simulink model "crazyflie"  (R2023a)
settings: Solver=FixedStepDiscrete  StartTime=0.0  StopTime=160  FixedStep=0.001  RelTol=1e-3
undefined symbols (not defined in the file or in its folder): K
settings Model: PauseTimes=7  Creator=Zrean  LastModifiedBy=mosta
settings SolverCC: AlgebraicLoopSolver=TrustRegion
settings DataIOCC: ReturnWorkspaceOutputs=off
settings OptimizationCC: DefaultParameterBehavior=Inlined  UseDivisionForNetSlopeComputation=on  UseFloatMulNetSlope=on  UseSpecifiedMinMax=on  InlineInvariantSignals=on  PassReuseOutputArgsAs=Individual arguments  ZeroExternalMemoryAtStartup=off  ZeroInternalMemoryAtStartup=off  NoFixptDivByZeroProtection=on  EfficientFloat2IntCast=on  LifeSpan=1  EfficientTunableParamExpr=on
settings DebuggingCC: AlgebraicLoopMsg=error  ParameterTunabilityLossMsg=error  UnconnectedInputMsg=warning  UnconnectedOutputMsg=warning  UnconnectedLineMsg=warning  ArithmeticOperatorsInVariantConditions=warning
settings HardwareCC: ProdBitPerPointer=32  ProdBitPerSizeT=32  ProdBitPerPtrDiffT=32  ProdLargestAtomicInteger=Long  ProdLargestAtomicFloat=Double  ProdWordSize=32  ProdHWDeviceType=ARM Compatible->ARM Cortex
settings ModelReferenceCC: EnableRefExpFcnMdlSchedulingChecks=on
settings SFSimCC: SimUseLocalCustomCode=off  MATLABDynamicMemAlloc=off  CustomCodeUndefinedFunction=UseInterfaceOnly
settings RTWCC: Description=Embedded Coder  SystemTargetFile=ert.tlc  GenCodeOnly=on  TemplateMakefile=ert_default_tmf  GenerateReport=on  RTWUseLocalCustomCode=off  BuildConfiguration=Faster Runs  IncludeHyperlinkInReport=on  LaunchReport=on  GenerateTraceInfo=on  GenerateTraceReport=on  GenerateTraceReportSl=on  GenerateTraceReportSf=on  GenerateTraceReportEml=on  GenerateCodeMetricsReport=on
settings CodeAppCC: ForceParamTrailComments=on  IgnoreCustomStorageClasses=off  OperatorAnnotations=on  SimulinkDataObjDesc=on  SFDataObjDesc=on  MATLABFcnDesc=on  InsertBlockDesc=on  StateflowObjectComments=on  MATLABSourceComments=on
settings ERTTargetCC: TargetLangStandard=C99 (ISO)  MultiwordLength=2048  CombineSignalStateStructs=on  SuppressErrorStatus=on  SupportAbsoluteTime=off  SupportNonFinite=off  SupportComplex=off  InlinedParameterPlacement=NonHierarchical  ERTCustomFileTemplate=crazyflie_wrapper.tlc  ERTFilePackagingFormat=CompactWithDataFile
settings SimscapeCC: SimscapeNormalizeSystem=off

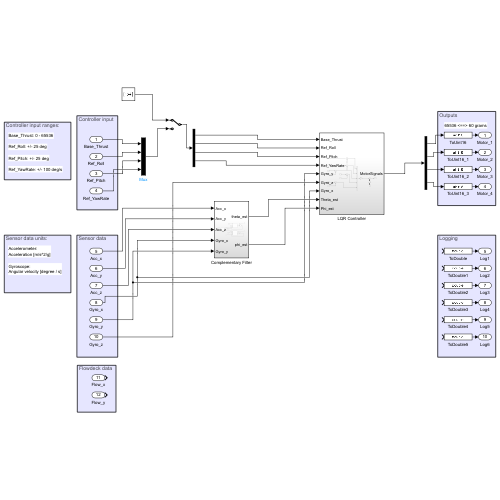
[thumbnail: Simulink's stored preview of the top-level diagram]
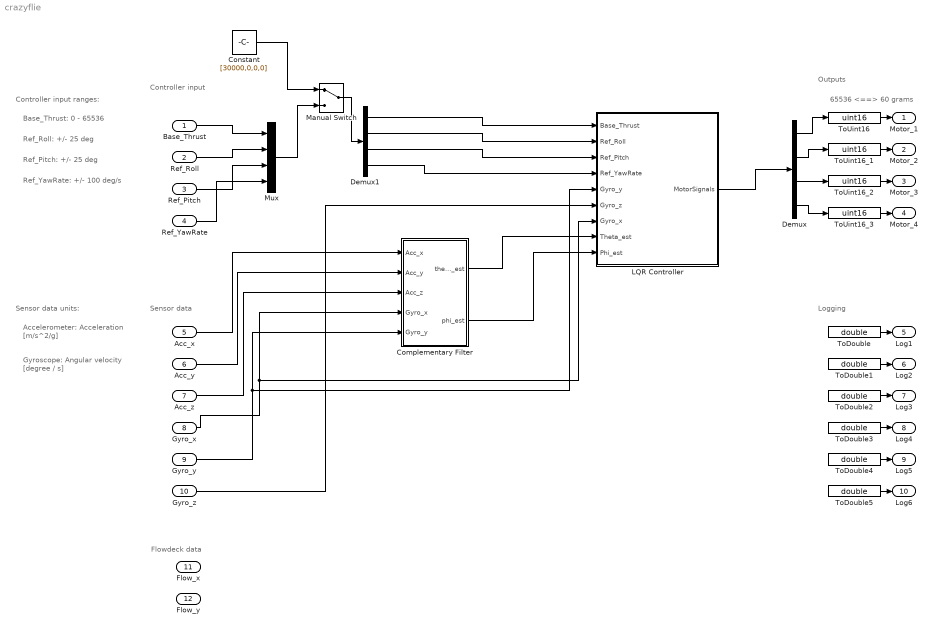
== system crazyflie ==
  note: 65536 <==> 60 grams
  note: Logging
  note: Outputs
  note: Sensor data
  note: Controller input
  note: Ref_Roll: +/- 25 deg
  note: Base_Thrust: 0 - 65536
  note: Ref_Pitch: +/- 25 deg
  note: Ref_YawRate: +/- 100 deg/s
  note: Controller input ranges:
  note: Gyroscope:
      | Angular velocity [degree / s]
  note: Accelerometer:
      | Acceleration [m/s^2/g]
  note: Sensor data units:
  note: Flowdeck data
  Base_Thrust : Inport  OutDataTypeStr=double
  Ref_Roll : Inport  Port=2  OutDataTypeStr=double
  Ref_Pitch : Inport  Port=3  OutDataTypeStr=double
  Ref_YawRate : Inport  Port=4  OutDataTypeStr=double
  Acc_x : Inport  Port=5  OutDataTypeStr=double  PortDimensions=1
  Acc_y : Inport  Port=6  OutDataTypeStr=double  PortDimensions=1
  Acc_z : Inport  Port=7  OutDataTypeStr=double  PortDimensions=1
  Gyro_x : Inport  Port=8  OutDataTypeStr=double  PortDimensions=1
  Gyro_y : Inport  Port=9  OutDataTypeStr=double  PortDimensions=1
  Gyro_z : Inport  Port=10  OutDataTypeStr=double  PortDimensions=1
  Flow_x : Inport  Port=11  OutDataTypeStr=int16  PortDimensions=1
  Flow_y : Inport  Port=12  OutDataTypeStr=int16  PortDimensions=1
  Complementary Filter : Subsystem
  Constant : Constant  Value=[30000,0,0,0]
  Demux : Demux
  Demux1 : Demux
  LQR Controller : Subsystem
  Manual Switch : ManualSwitch
  Mux : Mux
  ToDouble{,1..5} (6 alike) : DataTypeConversion  OutDataTypeStr=double  RndMeth=Floor
  ToUint16 : DataTypeConversion  OutDataTypeStr=uint16  RndMeth=Floor
  ToUint16_1 : DataTypeConversion  OutDataTypeStr=uint16  RndMeth=Floor
  ToUint16_2 : DataTypeConversion  OutDataTypeStr=uint16  RndMeth=Floor
  ToUint16_3 : DataTypeConversion  OutDataTypeStr=uint16  RndMeth=Floor
  Motor_1 : Outport  OutDataTypeStr=uint16  VectorParamsAs1DForOutWhenUnconnected=off  LockScale=on
  Motor_2 : Outport  Port=2  OutDataTypeStr=uint16  VectorParamsAs1DForOutWhenUnconnected=off  LockScale=on
  Motor_3 : Outport  Port=3  OutDataTypeStr=uint16  VectorParamsAs1DForOutWhenUnconnected=off  LockScale=on
  Motor_4 : Outport  Port=4  OutDataTypeStr=uint16  VectorParamsAs1DForOutWhenUnconnected=off  LockScale=on
  Log1 : Outport  Port=5  OutDataTypeStr=double  VectorParamsAs1DForOutWhenUnconnected=off
  Log2 : Outport  Port=6  OutDataTypeStr=double  VectorParamsAs1DForOutWhenUnconnected=off
  Log3 : Outport  Port=7  OutDataTypeStr=double  VectorParamsAs1DForOutWhenUnconnected=off
  Log4 : Outport  Port=8  OutDataTypeStr=double  VectorParamsAs1DForOutWhenUnconnected=off
  Log5 : Outport  Port=9  OutDataTypeStr=double  VectorParamsAs1DForOutWhenUnconnected=off
  Log6 : Outport  Port=10  OutDataTypeStr=double  VectorParamsAs1DForOutWhenUnconnected=off
  wires:
  ToUint16/1 -> Motor_1/1
  ToUint16_1/1 -> Motor_2/1
  ToUint16_2/1 -> Motor_3/1
  ToUint16_3/1 -> Motor_4/1
  ToDouble/1 -> Log1/1
  ToDouble1/1 -> Log2/1
  ToDouble2/1 -> Log3/1
  ToDouble3/1 -> Log4/1
  ToDouble4/1 -> Log5/1
  ToDouble5/1 -> Log6/1
  Acc_x/1 -> Complementary Filter/1(Acc_x)
  Acc_y/1 -> Complementary Filter/2(Acc_y)
  Acc_z/1 -> Complementary Filter/3(Acc_z)
  Gyro_x/1 -> LQR Controller/7(Gyro_x), Complementary Filter/4(Gyro_x)
  Gyro_y/1 -> LQR Controller/5(Gyro_y), Complementary Filter/5(Gyro_y)
  Demux/1 -> ToUint16/1
  Demux/2 -> ToUint16_1/1
  Demux/3 -> ToUint16_2/1
  Demux/4 -> ToUint16_3/1
  Complementary Filter/2(phi_est) -> LQR Controller/9(Phi_est)
  Complementary Filter/1(theta_est) -> LQR Controller/8(Theta_est)
  Gyro_z/1 -> LQR Controller/6(Gyro_z)
  LQR Controller/1(MotorSignals) -> Demux/1
  Demux1/1 -> LQR Controller/1(Base_Thrust)
  Demux1/2 -> LQR Controller/2(Ref_Roll)
  Demux1/3 -> LQR Controller/3(Ref_Pitch)
  Demux1/4 -> LQR Controller/4(Ref_YawRate)
  Constant/1 -> Manual Switch/1
  Manual Switch/1 -> Demux1/1
  Base_Thrust/1 -> Mux/1
  Ref_Roll/1 -> Mux/2
  Ref_Pitch/1 -> Mux/3
  Ref_YawRate/1 -> Mux/4
  Mux/1 -> Manual Switch/2

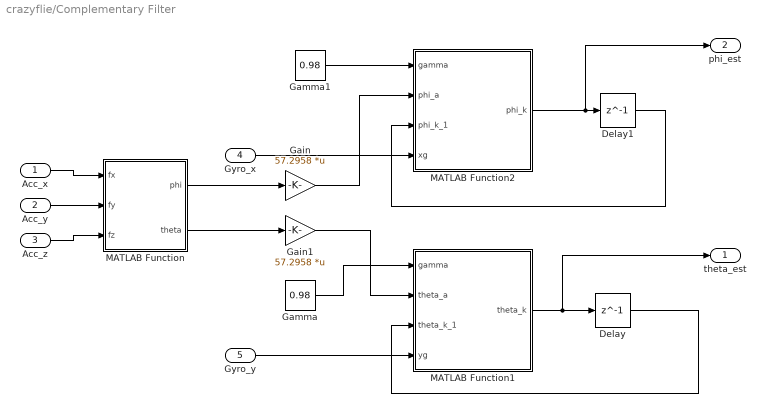
== system crazyflie/Complementary Filter ==
  Acc_x : Inport
  Acc_y : Inport  Port=2
  Acc_z : Inport  Port=3
  Gyro_x : Inport  Port=4
  Gyro_y : Inport  Port=5
  Delay : Delay  DelayLength=1
  Delay1 : Delay  DelayLength=1
  Gain : Gain  Gain=57.2958  Multiplication=Matrix(K*u)
  Gain1 : Gain  Gain=57.2958  Multiplication=Matrix(K*u)
  Gamma : Constant  Value=0.98
  Gamma1 : Constant  Value=0.98
  MATLAB Function : MATLAB Function  TreatAsAtomicUnit=on
  MATLAB Function1 : MATLAB Function  TreatAsAtomicUnit=on
  MATLAB Function2 : MATLAB Function  TreatAsAtomicUnit=on
  theta_est : Outport
  phi_est : Outport  Port=2
  wires:
  Delay1/1 -> MATLAB Function2/3(phi_k_1)
  Delay/1 -> MATLAB Function1/3(theta_k_1)
  Gamma/1 -> MATLAB Function1/1(gamma)
  MATLAB Function/2(theta) -> Gain1/1
  Gyro_x/1 -> MATLAB Function2/4(xg)
  Gamma1/1 -> MATLAB Function2/1(gamma)
  MATLAB Function/1(phi) -> Gain/1
  Gyro_y/1 -> MATLAB Function1/4(yg)
  Acc_x/1 -> MATLAB Function/1(fx)
  Acc_z/1 -> MATLAB Function/3(fz)
  Acc_y/1 -> MATLAB Function/2(fy)
  MATLAB Function2/1(phi_k) -> phi_est/1, Delay1/1
  MATLAB Function1/1(theta_k) -> theta_est/1, Delay/1
  Gain/1 -> MATLAB Function2/2(phi_a)
  Gain1/1 -> MATLAB Function1/2(theta_a)

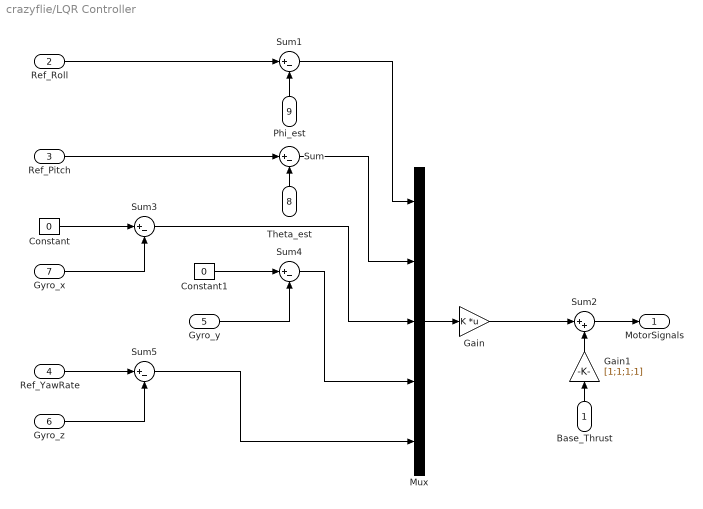
== system crazyflie/LQR Controller ==
  Base_Thrust : Inport
  Ref_Roll : Inport  Port=2
  Ref_Pitch : Inport  Port=3
  Ref_YawRate : Inport  Port=4
  Gyro_y : Inport  Port=5
  Gyro_z : Inport  Port=6
  Gyro_x : Inport  Port=7
  Theta_est : Inport  Port=8
  Phi_est : Inport  Port=9
  Constant : Constant  Value=0
  Constant1 : Constant  Value=0
  Gain : Gain  Gain=K  Multiplication=Matrix(K*u)
  Gain1 : Gain  Gain=[1;1;1;1]
  Mux : Mux  Inputs=5
  Sum{,1,3..5} (5 alike) : Sum  Inputs=|+-
  Sum2 : Sum  Inputs=|++
  MotorSignals : Outport
  wires:
  Sum/1 -> Mux/2
  Gain1/1 -> Sum2/2
  Theta_est/1 -> Sum/2
  Sum4/1 -> Mux/4
  Ref_Roll/1 -> Sum1/1
  Gain/1 -> Sum2/1
  Gyro_x/1 -> Sum3/2
  Sum1/1 -> Mux/1
  Sum5/1 -> Mux/5
  Constant1/1 -> Sum4/1
  Ref_Pitch/1 -> Sum/1
  Sum3/1 -> Mux/3
  Constant/1 -> Sum3/1
  Gyro_y/1 -> Sum4/2
  Gyro_z/1 -> Sum5/2
  Mux/1 -> Gain/1
  Base_Thrust/1 -> Gain1/1
  Phi_est/1 -> Sum1/2
  Ref_YawRate/1 -> Sum5/1
  Sum2/1 -> MotorSignals/1

== matlab function crazyflie/Complementary Filter/MATLAB Function1 ==
  data: gamma input; theta_k output; theta_a input; theta_k_1 input; yg input
function theta_k = fcn(gamma, theta_a,theta_k_1,yg)

theta_k = (1-gamma)*theta_a+gamma*(theta_k_1+0.001*yg);
end

== matlab function crazyflie/Complementary Filter/MATLAB Function ==
  data: fx input; phi output; fy input; fz input; theta output
function [phi,theta] = fcn(fx,fy,fz)

phi = atan2(fy,fz);
theta=atan2(-fx,sqrt(fy^2+fz^2));
end

== matlab function crazyflie/Complementary Filter/MATLAB Function2 ==
  data: gamma input; phi_k output; phi_a input; phi_k_1 input; xg input
function phi_k = fcn(gamma, phi_a,phi_k_1,xg)

phi_k = (1-gamma)*phi_a+gamma*(phi_k_1+0.001*xg);
end
